simulink model "Closed_loop_Model"  (R2024b)
settings: Solver=VariableStepAuto  StartTime=0.0  StopTime=10.0  RelTol=1e-3
settings Model: Creator=Zohaib  LastModifiedBy=Zohaib

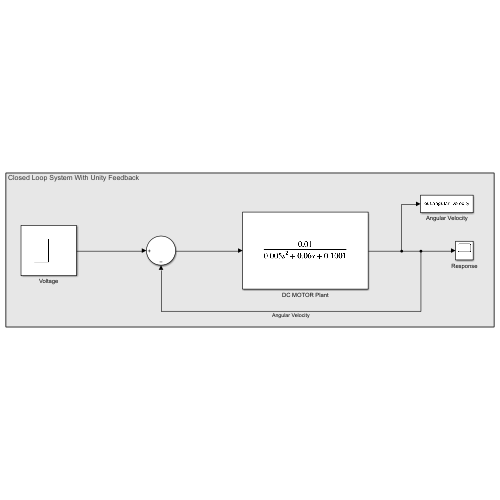
[thumbnail: Simulink's stored preview of the top-level diagram]
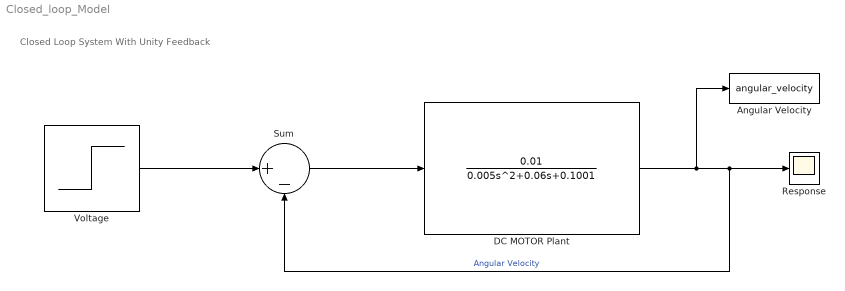
== system Closed_loop_Model ==
  note: Closed Loop System With Unity Feedback
  Angular Velocity : ToWorkspace  VariableName=angular_velocity  SaveFormat=Timeseries  SampleTime=-1
  DC MOTOR Plant : TransferFcn  Numerator=[0.01]  Denominator="[0.005  0.06  0.1001]"
  Response : Scope
  Sum : Sum  Inputs=|+-
  Voltage : Step  SampleTime=0
  wires:
  Sum/1 -> DC MOTOR Plant/1
  DC MOTOR Plant/1 -> Angular Velocity/1, Response/1, Sum/2  "Angular Velocity"
  Voltage/1 -> Sum/1
